simulink model "Hydroelectric"  (R2024b)
settings: Solver=VariableStepAuto  StartTime=0.0  StopTime=2000  RelTol=1e-3
settings Model: Creator=aspar  LastModifiedBy=aspar

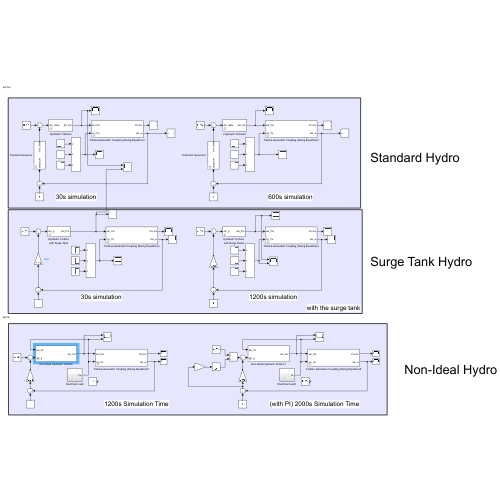
[thumbnail: Simulink's stored preview of the top-level diagram]
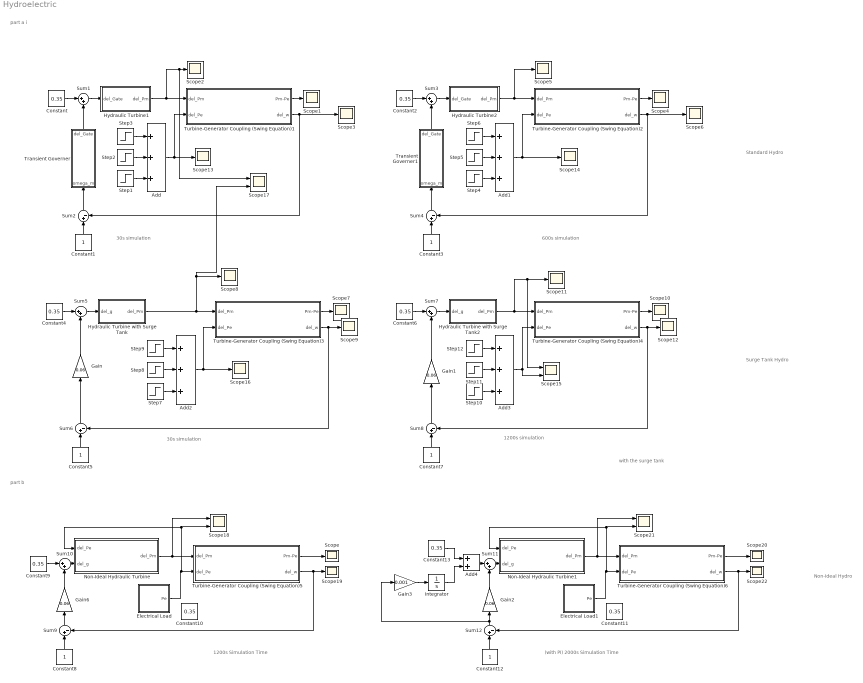
== system Hydroelectric ==
  note: (with PI) 2000s Simulation Time
  note: part b
  note: with the surge tank
  note: part a i
  note: 30s simulation
  note: 600s simulation
  note: 30s simulation
  note: 1200s simulation
  note: 1200s Simulation Time
  note: Standard Hydro
  note: Surge Tank Hydro
  note: Non-Ideal Hydro
  Add{,1..3} (4 alike) : Sum  Inputs=+++
  Add4 : Sum
  Constant{,2,4,6,9..11,13} (8 alike) : Constant  Value=0.35
  Constant{1,3,5,7..8,12} (6 alike) : Constant
  Electrical Load : Subsystem
  Electrical Load1 : Subsystem
  Gain{,1..2,6} (4 alike) : Gain  Gain=0.06
  Gain3 : Gain  Gain=0.001
  Hydraulic Turbine with Surge Tank : Subsystem  mask{T_w=2.6, w_n=1.53846, ini=0.35}
  Hydraulic Turbine with Surge Tank2 : Subsystem  mask{T_w=2.6, w_n=1.53846, ini=0.35}
  Hydraulic Turbine1 : Subsystem  mask{Tw=2.6, init1=0.35}
  Hydraulic Turbine2 : Subsystem  mask{Tw=2.6, init1=0.35}
  Integrator : Integrator
  Non-Ideal Hydraulic Turbine : Subsystem  mask{T_omega=2.6}
  Non-Ideal Hydraulic Turbine1 : Subsystem  mask{T_omega=2.6}
  Scope{,1..14,16,19..20,22} (19 alike) : Scope
  Scope{15,17..18,21} (4 alike) : Scope  NumInputPorts=2
  Step1 : Step  Time=15  After=0.5  SampleTime=0
  Step10 : Step  Time=900  After=0.5  SampleTime=0
  Step11 : Step  Time=600  After=-0.2  SampleTime=0
  Step12 : Step  Time=300  Before=0.35  After=0.6  SampleTime=0
  Step2 : Step  Time=10  After=-0.2  SampleTime=0
  Step3 : Step  Time=5  Before=0.35  After=0.6  SampleTime=0
  Step4 : Step  Time=450  After=0.5  SampleTime=0
  Step5 : Step  Time=300  After=-0.2  SampleTime=0
  Step6 : Step  Time=150  Before=0.35  After=0.6  SampleTime=0
  Step7 : Step  Time=15  After=0.5  SampleTime=0
  Step8 : Step  Time=10  After=-0.2  SampleTime=0
  Step9 : Step  Time=5  Before=0.35  After=0.6  SampleTime=0
  Sum{1,3,5,7,10..11} (6 alike) : Sum  Inputs=|++
  Sum{2,4,6,8..9,12} (6 alike) : Sum  Inputs=|+-
  Transient Governer : Subsystem  mask{Tr=10.4, R=0.06, delta=1.5757576, init2=0}
  Transient Governer1 : Subsystem  mask{Tr=10.4, R=0.06, delta=1.5757576, init2=0}
  Turbine-Generator Coupling (Swing Equation)1 : Subsystem  mask{H=3.3, w_ini=1, D=0}
  Turbine-Generator Coupling (Swing Equation)2 : Subsystem  mask{H=3.3, w_ini=1, D=0}
  Turbine-Generator Coupling (Swing Equation)3 : Subsystem  mask{H=3.3, w_ini=1, D=0}
  Turbine-Generator Coupling (Swing Equation)4 : Subsystem  mask{H=3.3, w_ini=1, D=0}
  Turbine-Generator Coupling (Swing Equation)5 : Subsystem  mask{H=3.3, w_ini=1, D=0}
  Turbine-Generator Coupling (Swing Equation)6 : Subsystem  mask{H=3.3, w_ini=1, D=0}
  wires:
  Sum1/1 -> Hydraulic Turbine1/1(del_Gate)
  Turbine-Generator Coupling (Swing Equation)1/2(del_w) -> Sum2/2, Scope3/1
  Turbine-Generator Coupling (Swing Equation)1/1(Pm-Pe) -> Scope1/1
  Hydraulic Turbine1/1(del_Pm) -> Scope17/1, Scope2/1, Turbine-Generator Coupling (Swing Equation)1/1(del_Pm)
  Constant/1 -> Sum1/1
  Transient Governer/1(del_Gate) -> Sum1/2
  Add/1 -> Scope13/1, Turbine-Generator Coupling (Swing Equation)1/2(del_Pe)
  Step1/1 -> Add/3
  Step2/1 -> Add/2
  Step3/1 -> Add/1
  Sum2/1 -> Transient Governer/1(omega_m)
  Constant1/1 -> Sum2/1
  Constant3/1 -> Sum4/1
  Sum4/1 -> Transient Governer1/1(omega_m)
  Turbine-Generator Coupling (Swing Equation)2/2(del_w) -> Sum4/2, Scope6/1
  Hydraulic Turbine2/1(del_Pm) -> Scope5/1, Turbine-Generator Coupling (Swing Equation)2/1(del_Pm)
  Step5/1 -> Add1/2
  Step4/1 -> Add1/3
  Turbine-Generator Coupling (Swing Equation)2/1(Pm-Pe) -> Scope4/1
  Step6/1 -> Add1/1
  Constant2/1 -> Sum3/1
  Add1/1 -> Scope14/1, Turbine-Generator Coupling (Swing Equation)2/2(del_Pe)
  Transient Governer1/1(del_Gate) -> Sum3/2
  Sum3/1 -> Hydraulic Turbine2/1(del_Gate)
  Constant5/1 -> Sum6/1
  Sum6/1 -> Gain/1
  Turbine-Generator Coupling (Swing Equation)3/2(del_w) -> Sum6/2, Scope9/1
  Hydraulic Turbine with Surge Tank/1(del_Pm) -> Scope17/2, Scope8/1, Turbine-Generator Coupling (Swing Equation)3/1(del_Pm)
  Step8/1 -> Add2/2
  Step7/1 -> Add2/3
  Turbine-Generator Coupling (Swing Equation)3/1(Pm-Pe) -> Scope7/1
  Step9/1 -> Add2/1
  Constant4/1 -> Sum5/1
  Add2/1 -> Scope16/1, Turbine-Generator Coupling (Swing Equation)3/2(del_Pe)
  Gain/1 -> Sum5/2
  Sum5/1 -> Hydraulic Turbine with Surge Tank/1(del_g)
  Gain1/1 -> Sum7/2
  Sum7/1 -> Hydraulic Turbine with Surge Tank2/1(del_g)
  Add3/1 -> Scope15/2, Turbine-Generator Coupling (Swing Equation)4/2(del_Pe)
  Turbine-Generator Coupling (Swing Equation)4/2(del_w) -> Sum8/2, Scope12/1
  Step11/1 -> Add3/2
  Constant6/1 -> Sum7/1
  Step12/1 -> Add3/1
  Hydraulic Turbine with Surge Tank2/1(del_Pm) -> Scope15/1, Scope11/1, Turbine-Generator Coupling (Swing Equation)4/1(del_Pm)
  Constant7/1 -> Sum8/1
  Turbine-Generator Coupling (Swing Equation)4/1(Pm-Pe) -> Scope10/1
  Sum8/1 -> Gain1/1
  Step10/1 -> Add3/3
  Non-Ideal Hydraulic Turbine/1(del_Pm) -> Scope18/1, Turbine-Generator Coupling (Swing Equation)5/1(del_Pm)
  Turbine-Generator Coupling (Swing Equation)5/1(Pm-Pe) -> Scope/1
  Sum9/1 -> Gain6/1
  Constant8/1 -> Sum9/1
  Turbine-Generator Coupling (Swing Equation)5/2(del_w) -> Scope19/1, Sum9/2
  Constant9/1 -> Sum10/1
  Sum10/1 -> Non-Ideal Hydraulic Turbine/2(del_g)
  Gain6/1 -> Sum10/2
  Electrical Load/1(Pe) -> Non-Ideal Hydraulic Turbine/1(del_Pe), Scope18/2, Turbine-Generator Coupling (Swing Equation)5/2(del_Pe)
  Sum11/1 -> Non-Ideal Hydraulic Turbine1/2(del_g)
  Electrical Load1/1(Pe) -> Non-Ideal Hydraulic Turbine1/1(del_Pe), Scope21/2, Turbine-Generator Coupling (Swing Equation)6/2(del_Pe)
  Gain2/1 -> Sum11/2
  Add4/1 -> Sum11/1
  Turbine-Generator Coupling (Swing Equation)6/1(Pm-Pe) -> Scope20/1
  Constant12/1 -> Sum12/1
  Sum12/1 -> Gain3/1, Gain2/1
  Non-Ideal Hydraulic Turbine1/1(del_Pm) -> Scope21/1, Turbine-Generator Coupling (Swing Equation)6/1(del_Pm)
  Turbine-Generator Coupling (Swing Equation)6/2(del_w) -> Scope22/1, Sum12/2
  Integrator/1 -> Add4/2
  Constant13/1 -> Add4/1
  Gain3/1 -> Integrator/1

== system Hydroelectric/Electrical Load ==
  Add5 : Sum  Inputs=+++
  Step13 : Step  Time=900  After=0.5  SampleTime=0
  Step14 : Step  Time=600  After=-0.2  SampleTime=0
  Step15 : Step  Time=300  Before=0.35  After=0.6  SampleTime=0
  Pe : Outport
  wires:
  Step15/1 -> Add5/1
  Add5/1 -> Pe/1
  Step13/1 -> Add5/3
  Step14/1 -> Add5/2

== system Hydroelectric/Electrical Load1 ==
  Add5 : Sum  Inputs=+++
  Step13 : Step  Time=900  After=0.5  SampleTime=0
  Step14 : Step  Time=600  After=-0.2  SampleTime=0
  Step15 : Step  Time=300  Before=0.35  After=0.6  SampleTime=0
  Pe : Outport
  wires:
  Step15/1 -> Add5/1
  Add5/1 -> Pe/1
  Step13/1 -> Add5/3
  Step14/1 -> Add5/2

== system Hydroelectric/Hydraulic Turbine with Surge Tank ==
  del_g : Inport
  Constant : Constant  Value=ini
  Sum : Sum  Inputs=|+-
  Sum1 : Sum  Inputs=|++
  Transfer Fcn : TransferFcn  Numerator=[(1/w_n)^2 -T_w 1]  Denominator=[(1/w_n)^2 0.5*T_w 1]
  del_Pm : Outport
  wires:
  Sum/1 -> Transfer Fcn/1
  del_g/1 -> Sum/1
  Transfer Fcn/1 -> Sum1/1
  Sum1/1 -> del_Pm/1
  Constant/1 -> Sum1/2, Sum/2

== system Hydroelectric/Hydraulic Turbine with Surge Tank2 ==
  del_g : Inport
  Constant : Constant  Value=ini
  Sum : Sum  Inputs=|+-
  Sum1 : Sum  Inputs=|++
  Transfer Fcn : TransferFcn  Numerator=[(1/w_n)^2 -T_w 1]  Denominator=[(1/w_n)^2 0.5*T_w 1]
  del_Pm : Outport
  wires:
  Sum/1 -> Transfer Fcn/1
  del_g/1 -> Sum/1
  Transfer Fcn/1 -> Sum1/1
  Sum1/1 -> del_Pm/1
  Constant/1 -> Sum1/2, Sum/2

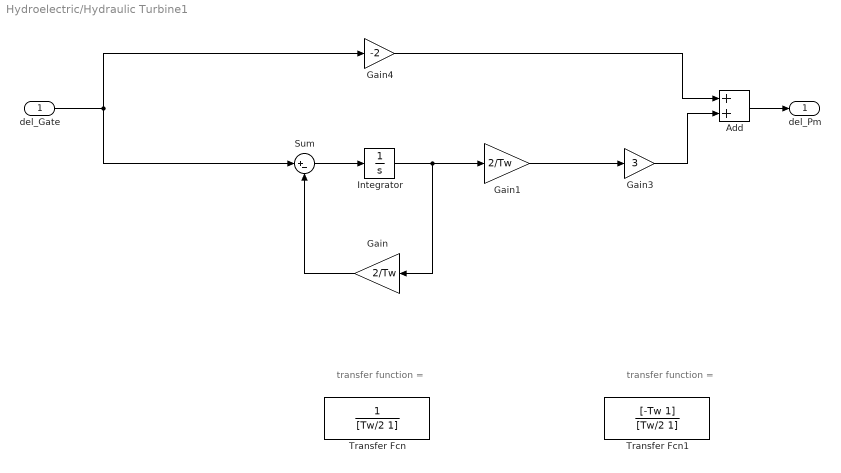
== system Hydroelectric/Hydraulic Turbine1 ==
  note: transfer function =
  note: transfer function =
  del_Gate : Inport
  Add : Sum
  Gain : Gain  Gain=2/Tw
  Gain1 : Gain  Gain=2/Tw
  Gain3 : Gain  Gain=3
  Gain4 : Gain  Gain=-2
  Integrator : Integrator  InitialCondition=(Tw*init1)/2
  Sum : Sum  Inputs=|+-
  Transfer Fcn : TransferFcn  Denominator=[Tw/2 1]
  Transfer Fcn1 : TransferFcn  Numerator=[-Tw 1]  Denominator=[Tw/2 1]
  del_Pm : Outport
  wires:
  Gain/1 -> Sum/2
  Integrator/1 -> Gain1/1, Gain/1
  Sum/1 -> Integrator/1
  del_Gate/1 -> Sum/1, Gain4/1
  Add/1 -> del_Pm/1
  Gain4/1 -> Add/1
  Gain1/1 -> Gain3/1
  Gain3/1 -> Add/2

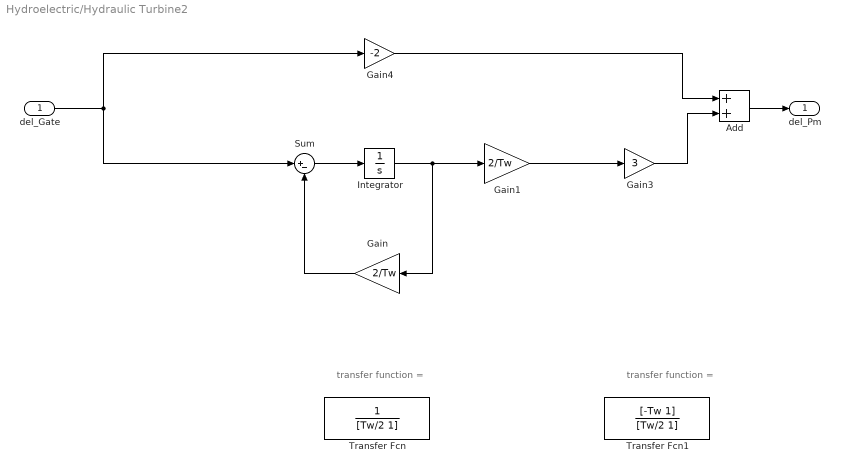
== system Hydroelectric/Hydraulic Turbine2 ==
  note: transfer function =
  note: transfer function =
  del_Gate : Inport
  Add : Sum
  Gain : Gain  Gain=2/Tw
  Gain1 : Gain  Gain=2/Tw
  Gain3 : Gain  Gain=3
  Gain4 : Gain  Gain=-2
  Integrator : Integrator  InitialCondition=(Tw*init1)/2
  Sum : Sum  Inputs=|+-
  Transfer Fcn : TransferFcn  Denominator=[Tw/2 1]
  Transfer Fcn1 : TransferFcn  Numerator=[-Tw 1]  Denominator=[Tw/2 1]
  del_Pm : Outport
  wires:
  Gain/1 -> Sum/2
  Integrator/1 -> Gain1/1, Gain/1
  Sum/1 -> Integrator/1
  del_Gate/1 -> Sum/1, Gain4/1
  Add/1 -> del_Pm/1
  Gain4/1 -> Add/1
  Gain1/1 -> Gain3/1
  Gain3/1 -> Add/2

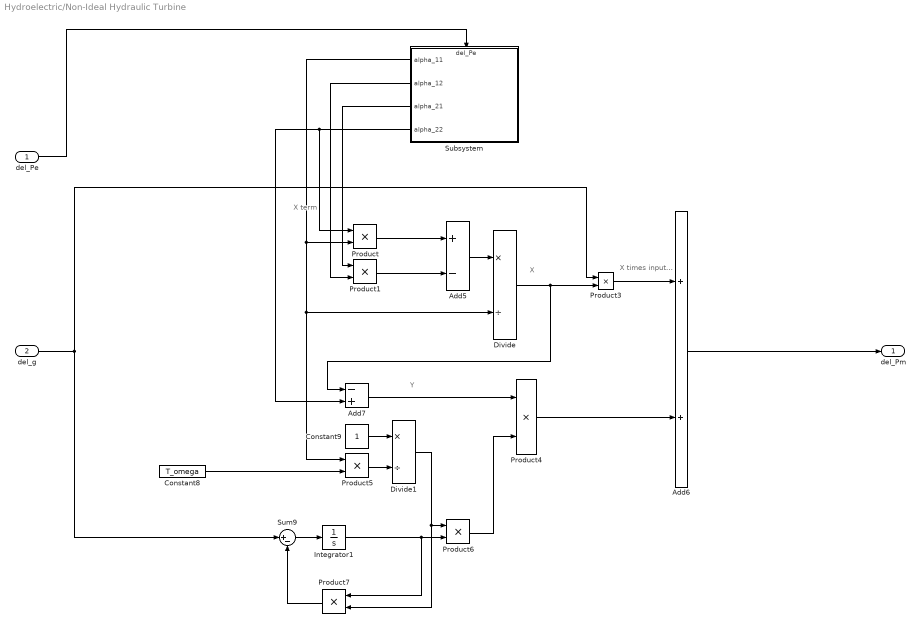
== system Hydroelectric/Non-Ideal Hydraulic Turbine ==
  note: Y
  note: X
  note: X times input...
  note: X term
  del_Pe : Inport
  del_g : Inport  Port=2
  Add5 : Sum  Inputs=+-
  Add6 : Sum
  Add7 : Sum  Inputs=-+
  Constant8 : Constant  Value=T_omega
  Constant9 : Constant
  Divide : Product  Inputs=*/
  Divide1 : Product  Inputs=*/
  Integrator1 : Integrator
  Product{,1,3..7} (7 alike) : Product
  Subsystem : Subsystem
      settings: PortSchema="{\"entries\":[{\"content\":{\"sides\":[{\"content\":{},\"type\":\"ConnectorPlacement.EquallySpacedRectSide\",\"uuid\":\"fe6d16d0-3695-435b-9d53-18f10f1c17de\"},{\"content\":{\"connectorIds\":[\"Out1\",\"Out2\",\"Out3\",\"Out4\"],\"side\":\"RIGHT\"},\"type\":\"ConnectorPlacement.EquallySpacedRectSide\",\"uuid\":\"00803313-5ddf-4c32-9044-1b4ef5a08615\"},{\"content\":{\"connectorIds\":[\"In1\"],\"side\":\"TOP\"},\"type\":\"ConnectorPlacement.EquallySpacedRectSide\",\"uuid\":\"b36d84d4-0dcd-458b-8f97-687f5ce90897\"}]},\"type\":\"ConnectorPlacement.EquallySpacedConnector\",\"uuid\":\"7d286004-7f8c-4cbb-b2bc-e5bc9d835532\"}],\"packageUris\":[\"http://schema.mathworks.com/mf0/Connector/R2020b\"],\"version\":\"1.0\"}"
  Sum9 : Sum  Inputs=|+-
  del_Pm : Outport
  wires:
  Product6/1 -> Product4/2
  Product1/1 -> Add5/2
  Divide1/1 -> Product7/2, Product6/1
  Product/1 -> Add5/1
  Integrator1/1 -> Product7/1, Product6/2
  Product5/1 -> Divide1/2
  Add7/1 -> Product4/1
  Subsystem/1(alpha_11) -> Product5/1, Divide/2, Product/2
  Product4/1 -> Add6/2
  Subsystem/4(alpha_22) -> Add7/2, Product/1
  Divide/1 -> Add7/1, Product3/2
  Constant8/1 -> Product5/2
  Subsystem/3(alpha_21) -> Product1/1
  Add5/1 -> Divide/1
  Sum9/1 -> Integrator1/1
  Subsystem/2(alpha_12) -> Product1/2
  Product7/1 -> Sum9/2
  del_Pe/1 -> Subsystem/1(del_Pe)
  del_g/1 -> Product3/1, Sum9/1
  Constant9/1 -> Divide1/1
  Product3/1 -> Add6/1
  Add6/1 -> del_Pm/1

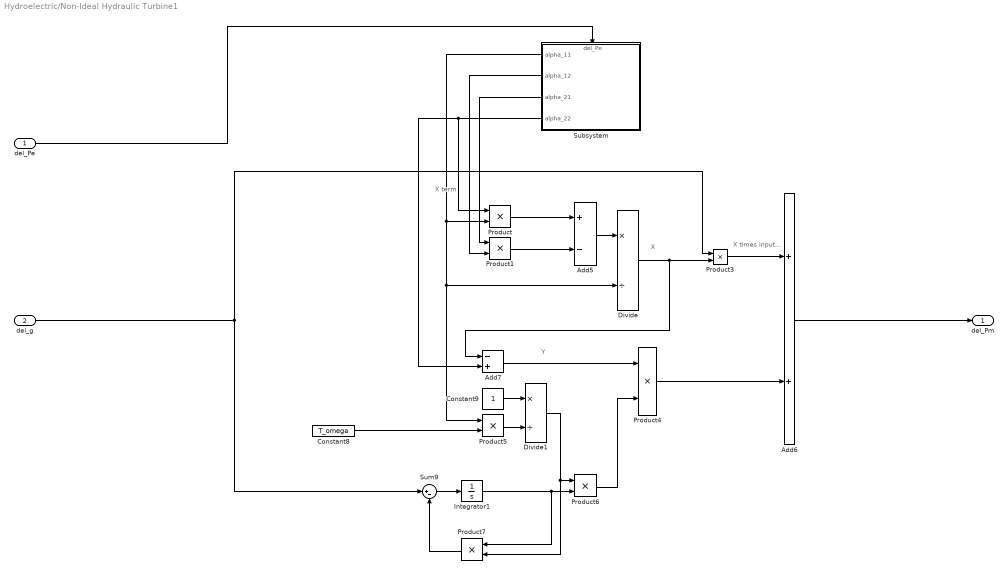
== system Hydroelectric/Non-Ideal Hydraulic Turbine1 ==
  note: Y
  note: X
  note: X times input...
  note: X term
  del_Pe : Inport
  del_g : Inport  Port=2
  Add5 : Sum  Inputs=+-
  Add6 : Sum
  Add7 : Sum  Inputs=-+
  Constant8 : Constant  Value=T_omega
  Constant9 : Constant
  Divide : Product  Inputs=*/
  Divide1 : Product  Inputs=*/
  Integrator1 : Integrator
  Product{,1,3..7} (7 alike) : Product
  Subsystem : Subsystem
      settings: PortSchema="{\"entries\":[{\"content\":{\"sides\":[{\"content\":{},\"type\":\"ConnectorPlacement.EquallySpacedRectSide\",\"uuid\":\"fe6d16d0-3695-435b-9d53-18f10f1c17de\"},{\"content\":{\"connectorIds\":[\"Out1\",\"Out2\",\"Out3\",\"Out4\"],\"side\":\"RIGHT\"},\"type\":\"ConnectorPlacement.EquallySpacedRectSide\",\"uuid\":\"00803313-5ddf-4c32-9044-1b4ef5a08615\"},{\"content\":{\"connectorIds\":[\"In1\"],\"side\":\"TOP\"},\"type\":\"ConnectorPlacement.EquallySpacedRectSide\",\"uuid\":\"b36d84d4-0dcd-458b-8f97-687f5ce90897\"}]},\"type\":\"ConnectorPlacement.EquallySpacedConnector\",\"uuid\":\"7d286004-7f8c-4cbb-b2bc-e5bc9d835532\"}],\"packageUris\":[\"http://schema.mathworks.com/mf0/Connector/R2020b\"],\"version\":\"1.0\"}"
  Sum9 : Sum  Inputs=|+-
  del_Pm : Outport
  wires:
  Product6/1 -> Product4/2
  Product1/1 -> Add5/2
  Divide1/1 -> Product7/2, Product6/1
  Product/1 -> Add5/1
  Integrator1/1 -> Product7/1, Product6/2
  Product5/1 -> Divide1/2
  Add7/1 -> Product4/1
  Subsystem/1(alpha_11) -> Product5/1, Divide/2, Product/2
  Product4/1 -> Add6/2
  Subsystem/4(alpha_22) -> Add7/2, Product/1
  Divide/1 -> Add7/1, Product3/2
  Constant8/1 -> Product5/2
  Subsystem/3(alpha_21) -> Product1/1
  Add5/1 -> Divide/1
  Sum9/1 -> Integrator1/1
  Subsystem/2(alpha_12) -> Product1/2
  Product7/1 -> Sum9/2
  del_Pe/1 -> Subsystem/1(del_Pe)
  del_g/1 -> Product3/1, Sum9/1
  Constant9/1 -> Divide1/1
  Product3/1 -> Add6/1
  Add6/1 -> del_Pm/1

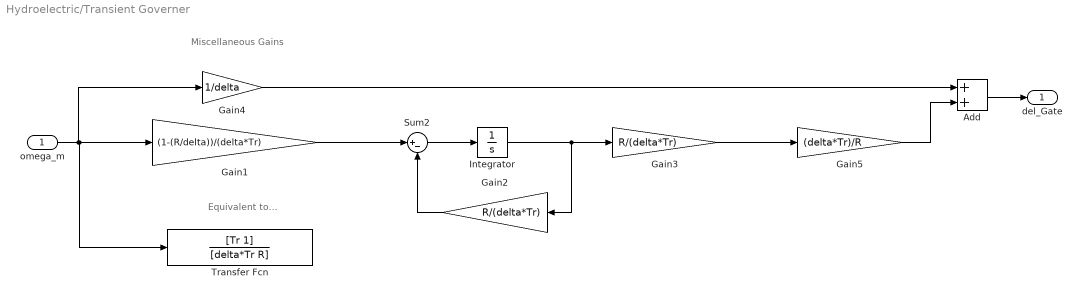
== system Hydroelectric/Transient Governer ==
  note: Miscellaneous Gains
  note: Equivalent to...
  omega_m : Inport
  Add : Sum
  Gain1 : Gain  Gain=(1-(R/delta))/(delta*Tr)
  Gain2 : Gain  Gain=R/(delta*Tr)
  Gain3 : Gain  Gain=R/(delta*Tr)
  Gain4 : Gain  Gain=1/delta
  Gain5 : Gain  Gain=(delta*Tr)/R
  Integrator : Integrator  InitialCondition=-Tr*init2/R%-Tr/R
  Sum2 : Sum  Inputs=|+-
  Transfer Fcn : TransferFcn  Numerator=[Tr 1]  Denominator=[delta*Tr R]
  del_Gate : Outport
  wires:
  Add/1 -> del_Gate/1
  Integrator/1 -> Gain3/1, Gain2/1
  omega_m/1 -> Gain4/1, Transfer Fcn/1, Gain1/1
  Gain1/1 -> Sum2/1
  Gain4/1 -> Add/1
  Sum2/1 -> Integrator/1
  Gain2/1 -> Sum2/2
  Gain3/1 -> Gain5/1
  Gain5/1 -> Add/2

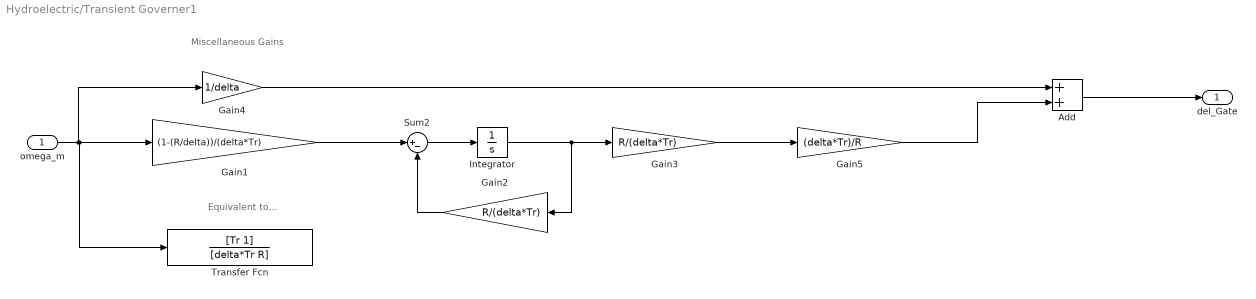
== system Hydroelectric/Transient Governer1 ==
  note: Miscellaneous Gains
  note: Equivalent to...
  omega_m : Inport
  Add : Sum
  Gain1 : Gain  Gain=(1-(R/delta))/(delta*Tr)
  Gain2 : Gain  Gain=R/(delta*Tr)
  Gain3 : Gain  Gain=R/(delta*Tr)
  Gain4 : Gain  Gain=1/delta
  Gain5 : Gain  Gain=(delta*Tr)/R
  Integrator : Integrator  InitialCondition=-Tr*init2/R%-Tr/R
  Sum2 : Sum  Inputs=|+-
  Transfer Fcn : TransferFcn  Numerator=[Tr 1]  Denominator=[delta*Tr R]
  del_Gate : Outport
  wires:
  Add/1 -> del_Gate/1
  Integrator/1 -> Gain3/1, Gain2/1
  omega_m/1 -> Gain4/1, Transfer Fcn/1, Gain1/1
  Gain1/1 -> Sum2/1
  Gain4/1 -> Add/1
  Sum2/1 -> Integrator/1
  Gain2/1 -> Sum2/2
  Gain3/1 -> Gain5/1
  Gain5/1 -> Add/2

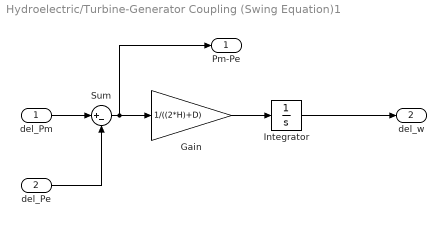
== system Hydroelectric/Turbine-Generator Coupling (Swing Equation)1 ==
  del_Pm : Inport
  del_Pe : Inport  Port=2
  Gain : Gain  Gain=1/((2*H)+D)
  Integrator : Integrator  InitialCondition=w_ini
  Sum : Sum  Inputs=|+-
  Pm-Pe : Outport
  del_w : Outport  Port=2
  wires:
  Gain/1 -> Integrator/1
  Sum/1 -> Pm-Pe/1, Gain/1
  del_Pm/1 -> Sum/1
  del_Pe/1 -> Sum/2
  Integrator/1 -> del_w/1

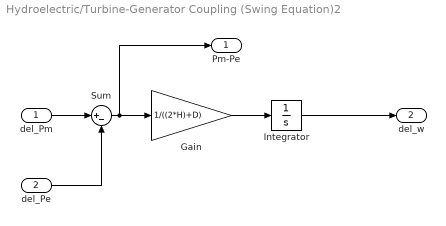
== system Hydroelectric/Turbine-Generator Coupling (Swing Equation)2 ==
  del_Pm : Inport
  del_Pe : Inport  Port=2
  Gain : Gain  Gain=1/((2*H)+D)
  Integrator : Integrator  InitialCondition=w_ini
  Sum : Sum  Inputs=|+-
  Pm-Pe : Outport
  del_w : Outport  Port=2
  wires:
  Gain/1 -> Integrator/1
  Sum/1 -> Pm-Pe/1, Gain/1
  del_Pm/1 -> Sum/1
  del_Pe/1 -> Sum/2
  Integrator/1 -> del_w/1

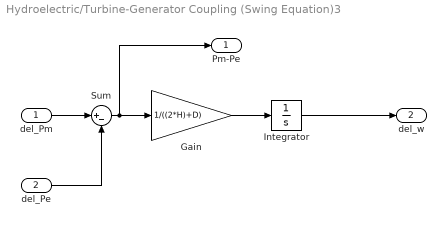
== system Hydroelectric/Turbine-Generator Coupling (Swing Equation)3 ==
  del_Pm : Inport
  del_Pe : Inport  Port=2
  Gain : Gain  Gain=1/((2*H)+D)
  Integrator : Integrator  InitialCondition=w_ini
  Sum : Sum  Inputs=|+-
  Pm-Pe : Outport
  del_w : Outport  Port=2
  wires:
  Gain/1 -> Integrator/1
  Sum/1 -> Pm-Pe/1, Gain/1
  del_Pm/1 -> Sum/1
  del_Pe/1 -> Sum/2
  Integrator/1 -> del_w/1

== system Hydroelectric/Turbine-Generator Coupling (Swing Equation)4 ==
  del_Pm : Inport
  del_Pe : Inport  Port=2
  Gain : Gain  Gain=1/((2*H)+D)
  Integrator : Integrator  InitialCondition=w_ini
  Sum : Sum  Inputs=|+-
  Pm-Pe : Outport
  del_w : Outport  Port=2
  wires:
  Gain/1 -> Integrator/1
  Sum/1 -> Pm-Pe/1, Gain/1
  del_Pm/1 -> Sum/1
  del_Pe/1 -> Sum/2
  Integrator/1 -> del_w/1

== system Hydroelectric/Turbine-Generator Coupling (Swing Equation)5 ==
  del_Pm : Inport
  del_Pe : Inport  Port=2
  Gain : Gain  Gain=1/((2*H)+D)
  Integrator : Integrator  InitialCondition=w_ini
  Sum : Sum  Inputs=|+-
  Pm-Pe : Outport
  del_w : Outport  Port=2
  wires:
  Gain/1 -> Integrator/1
  Sum/1 -> Pm-Pe/1, Gain/1
  del_Pm/1 -> Sum/1
  del_Pe/1 -> Sum/2
  Integrator/1 -> del_w/1

== system Hydroelectric/Turbine-Generator Coupling (Swing Equation)6 ==
  del_Pm : Inport
  del_Pe : Inport  Port=2
  Gain : Gain  Gain=1/((2*H)+D)
  Integrator : Integrator  InitialCondition=w_ini
  Sum : Sum  Inputs=|+-
  Pm-Pe : Outport
  del_w : Outport  Port=2
  wires:
  Gain/1 -> Integrator/1
  Sum/1 -> Pm-Pe/1, Gain/1
  del_Pm/1 -> Sum/1
  del_Pe/1 -> Sum/2
  Integrator/1 -> del_w/1

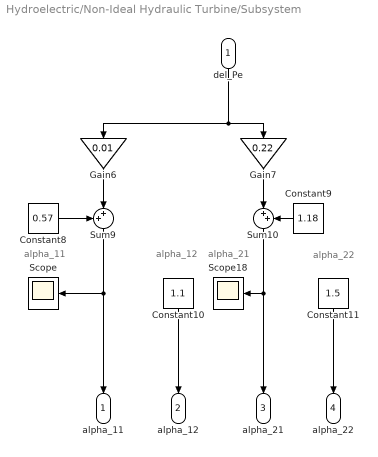
== system Hydroelectric/Non-Ideal Hydraulic Turbine/Subsystem ==
  note: alpha_11
  note: alpha_21
  note: alpha_12
  note: alpha_22
  del_Pe : Inport
  Constant10 : Constant  Value=1.1
  Constant11 : Constant  Value=1.5
  Constant8 : Constant  Value=0.57
  Constant9 : Constant  Value=1.18
  Gain6 : Gain  Gain=0.01
  Gain7 : Gain  Gain=0.22
  Scope : Scope
  Scope18 : Scope
  Sum10 : Sum  Inputs=|++
  Sum9 : Sum  Inputs=++|
  alpha_11 : Outport
  alpha_12 : Outport  Port=2
  alpha_21 : Outport  Port=3
  alpha_22 : Outport  Port=4
  wires:
  Sum9/1 -> alpha_11/1, Scope/1
  Constant11/1 -> alpha_22/1
  Sum10/1 -> alpha_21/1, Scope18/1
  del_Pe/1 -> Gain6/1, Gain7/1
  Constant10/1 -> alpha_12/1
  Constant8/1 -> Sum9/1
  Gain6/1 -> Sum9/2
  Constant9/1 -> Sum10/2
  Gain7/1 -> Sum10/1

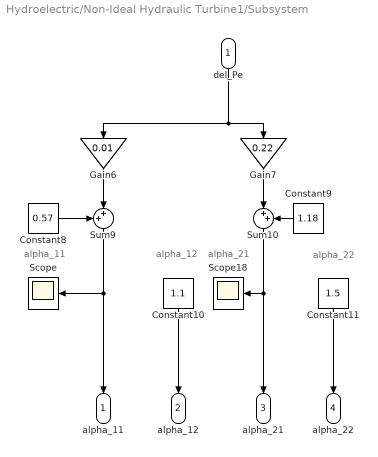
== system Hydroelectric/Non-Ideal Hydraulic Turbine1/Subsystem ==
  note: alpha_11
  note: alpha_21
  note: alpha_12
  note: alpha_22
  del_Pe : Inport
  Constant10 : Constant  Value=1.1
  Constant11 : Constant  Value=1.5
  Constant8 : Constant  Value=0.57
  Constant9 : Constant  Value=1.18
  Gain6 : Gain  Gain=0.01
  Gain7 : Gain  Gain=0.22
  Scope : Scope
  Scope18 : Scope
  Sum10 : Sum  Inputs=|++
  Sum9 : Sum  Inputs=++|
  alpha_11 : Outport
  alpha_12 : Outport  Port=2
  alpha_21 : Outport  Port=3
  alpha_22 : Outport  Port=4
  wires:
  Sum9/1 -> alpha_11/1, Scope/1
  Constant11/1 -> alpha_22/1
  Sum10/1 -> alpha_21/1, Scope18/1
  del_Pe/1 -> Gain6/1, Gain7/1
  Constant10/1 -> alpha_12/1
  Constant8/1 -> Sum9/1
  Gain6/1 -> Sum9/2
  Constant9/1 -> Sum10/2
  Gain7/1 -> Sum10/1
